simulink model "PMSM_ud_uq_regelung_BackUp"  (R2014b)
settings: Solver=ode4  StartTime=0.0  StopTime=0.2  FixedStep=5e-6  RelTol=1e-3
values from neighbouring files (symbols this model uses):
  f = 50    [parameter.mat]
  J = 0.00062    [parameter.mat]
  Ld = 0.000835    [parameter.mat]
  Lq = 0.000835    [parameter.mat]
  n_soll = 3000    [parameter.mat]
  p = 4    [parameter.mat]
  Psi_pm = 0.07147    [parameter.mat]
  R1 = 0.18    [parameter.mat]
settings Model: Creator=benjamin  LastModifiedBy=Benji

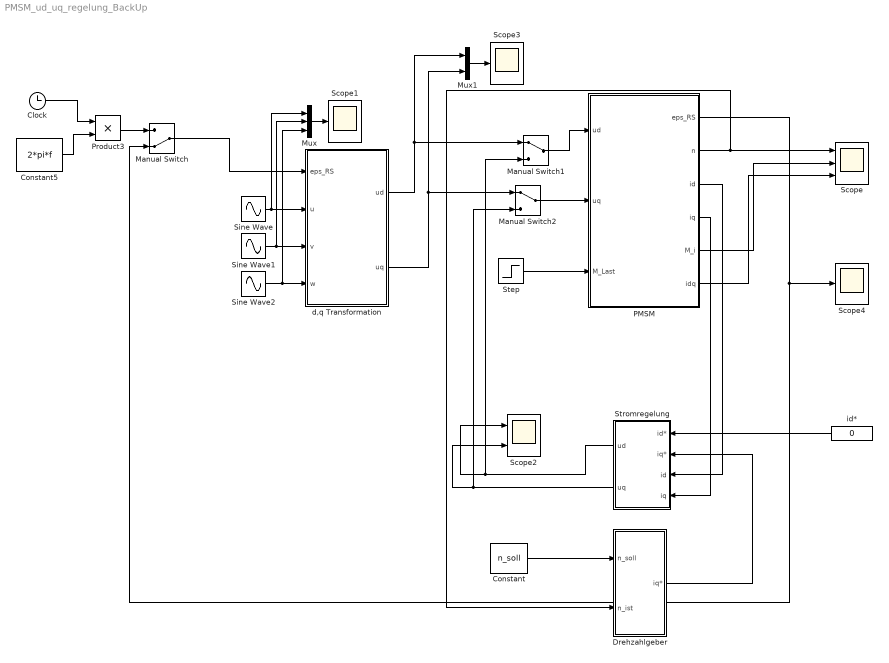
== system PMSM_ud_uq_regelung_BackUp ==
  Clock : Clock
  Constant : Constant  Value=n_soll
  Constant5 : Constant  Value=2*pi*f
  Drehzahlgeber : Subsystem
  Manual Switch : ManualSwitch  CurrentSetting=0
  Manual Switch1 : ManualSwitch
  Manual Switch2 : ManualSwitch
  Mux : Mux  Inputs=3
  Mux1 : Mux  Inputs=2
  PMSM : Subsystem
  Product3 : Product
  Scope : Scope  NumInputPorts=3
      settings: TimeRange=0.0108462013588635  YMin=0~-400~-800  YMax=1200~400~800  SaveName=ScopeData6
  Scope1 : Scope
      settings: TimeRange=0.2  YMin=-25000  YMax=20000
  Scope2 : Scope  NumInputPorts=2
      settings: TimeRange=0.2  YMin=-25000~-400  YMax=20000~400  SaveName=ScopeData2
  Scope3 : Scope
      settings: TimeRange=0.2  YMin=-25000  YMax=20000  SaveName=ScopeData3
  Scope4 : Scope
      settings: TimeRange=0.2  YMin=-25000  YMax=20000  SaveName=ScopeData4
  Sine Wave : Sin  Amplitude=230  Frequency=2*pi*f  SampleTime=0
  Sine Wave1 : Sin  Amplitude=230  Frequency=2*pi*f  Phase=(-2/3)*pi  SampleTime=0
  Sine Wave2 : Sin  Amplitude=230  Frequency=2*pi*f  Phase=(2/3)*pi  SampleTime=0
  Step : Step  Time=0.1  After=40  SampleTime=0
  Stromregelung : Subsystem
  d,q Transformation : Subsystem
  id* : Constant  Value=0
  wires:
  id*/1 -> Stromregelung/1(id*)
  Drehzahlgeber/1(iq*) -> Stromregelung/2(iq*)
  Constant/1 -> Drehzahlgeber/1(n_soll)
  PMSM/2(n) -> Drehzahlgeber/2(n_ist), Scope/1
  PMSM/5(M_i) -> Scope/2
  PMSM/6(idq) -> Scope/3
  Sine Wave/1 -> Mux/1, d,q Transformation/2(u)
  Sine Wave1/1 -> Mux/2, d,q Transformation/3(v)
  Sine Wave2/1 -> Mux/3, d,q Transformation/4(w)
  Mux/1 -> Scope1/1
  Stromregelung/1(ud) -> Scope2/1, Manual Switch1/2
  Stromregelung/2(uq) -> Scope2/2, Manual Switch2/2
  PMSM/3(id) -> Stromregelung/3(id)
  PMSM/4(iq) -> Stromregelung/4(iq)
  Mux1/1 -> Scope3/1
  d,q Transformation/1(ud) -> Manual Switch1/1, Mux1/1
  d,q Transformation/2(uq) -> Manual Switch2/1, Mux1/2
  Clock/1 -> Product3/1
  Constant5/1 -> Product3/2
  Product3/1 -> Manual Switch/1
  Manual Switch/1 -> d,q Transformation/1(eps_RS)
  PMSM/1(eps_RS) -> Scope4/1, Manual Switch/2
  Manual Switch1/1 -> PMSM/1("ud ")
  Manual Switch2/1 -> PMSM/2(uq)
  Step/1 -> PMSM/3(M_Last)

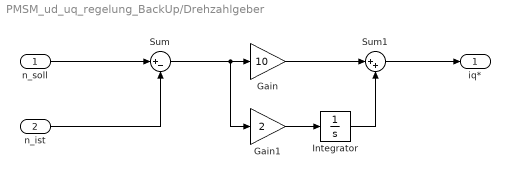
== system PMSM_ud_uq_regelung_BackUp/Drehzahlgeber ==
  n_soll : Inport
  n_ist : Inport  Port=2
  Gain : Gain  Gain=10
  Gain1 : Gain  Gain=2
  Integrator : Integrator
  Sum : Sum  Inputs=|+-
  Sum1 : Sum  Inputs=|++
  iq* : Outport
  wires:
  n_soll/1 -> Sum/1
  n_ist/1 -> Sum/2
  Sum/1 -> Gain1/1, Gain/1
  Gain/1 -> Sum1/1
  Gain1/1 -> Integrator/1
  Integrator/1 -> Sum1/2
  Sum1/1 -> iq*/1

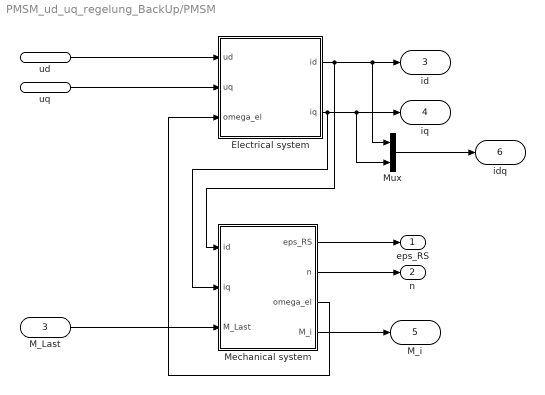
== system PMSM_ud_uq_regelung_BackUp/PMSM ==
  "ud " : Inport
  uq : Inport  Port=2
  M_Last : Inport  Port=3
  Electrical system : Subsystem
  Mechanical system : Subsystem
  Mux : Mux  Inputs=2
  eps_RS : Outport
  n : Outport  Port=2
  id : Outport  Port=3
  iq : Outport  Port=4
  M_i : Outport  Port=5
  idq : Outport  Port=6
  wires:
  Electrical system/1(id) -> Mux/1, id/1, Mechanical system/1(id)
  Electrical system/2(iq) -> Mux/2, iq/1, Mechanical system/2(iq)
  Mechanical system/3(omega_el) -> Electrical system/3(omega_el)
  Mechanical system/1(eps_RS) -> eps_RS/1
  Mechanical system/2(n) -> n/1
  Mechanical system/4(M_i) -> M_i/1
  M_Last/1 -> Mechanical system/3(M_Last)
  uq/1 -> Electrical system/2(uq)
  "ud "/1 -> Electrical system/1(ud)
  Mux/1 -> idq/1

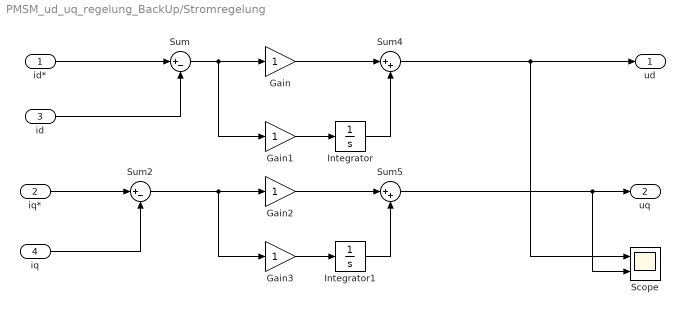
== system PMSM_ud_uq_regelung_BackUp/Stromregelung ==
  id* : Inport
  iq* : Inport  Port=2
  id : Inport  Port=3
  iq : Inport  Port=4
  Gain{,1..3} (4 alike) : Gain
  Integrator : Integrator
  Integrator1 : Integrator
  Scope : Scope  NumInputPorts=2
      settings: TimeRange=5  YMin=-1.3~-5  YMax=0~5
  Sum : Sum  Inputs=|+-
  Sum2 : Sum  Inputs=|+-
  Sum4 : Sum  Inputs=|++
  Sum5 : Sum  Inputs=|++
  ud : Outport
  uq : Outport  Port=2
  wires:
  Sum5/1 -> Scope/2, uq/1
  iq*/1 -> Sum2/1
  id*/1 -> Sum/1
  id/1 -> Sum/2
  iq/1 -> Sum2/2
  Sum4/1 -> ud/1, Scope/1
  Sum/1 -> Gain1/1, Gain/1
  Gain/1 -> Sum4/1
  Gain1/1 -> Integrator/1
  Integrator/1 -> Sum4/2
  Sum2/1 -> Gain3/1, Gain2/1
  Gain2/1 -> Sum5/1
  Gain3/1 -> Integrator1/1
  Integrator1/1 -> Sum5/2

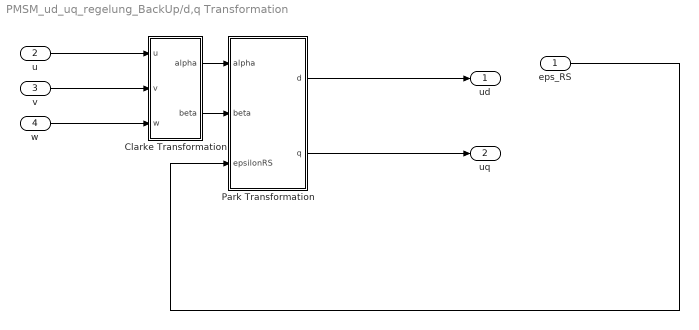
== system PMSM_ud_uq_regelung_BackUp/d,q Transformation ==
  eps_RS : Inport
  u : Inport  Port=2
  v : Inport  Port=3
  w : Inport  Port=4
  Clarke Transformation : Subsystem
  Park Transformation : Subsystem
  ud : Outport
  uq : Outport  Port=2
  wires:
  eps_RS/1 -> Park Transformation/3(epsilonRS)
  Clarke Transformation/1(alpha) -> Park Transformation/1(alpha)
  Clarke Transformation/2(beta) -> Park Transformation/2(beta)
  Park Transformation/1(d) -> ud/1
  Park Transformation/2(q) -> uq/1
  v/1 -> Clarke Transformation/2(v)
  u/1 -> Clarke Transformation/1(u)
  w/1 -> Clarke Transformation/3(w)

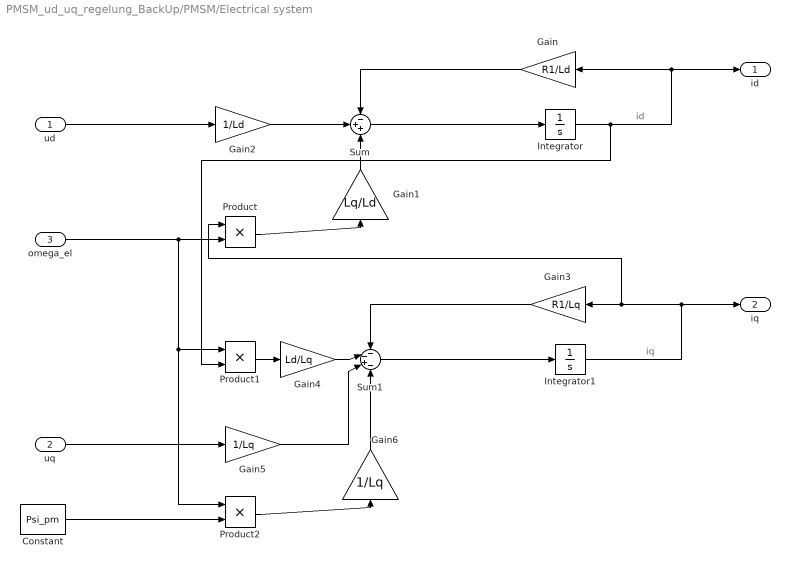
== system PMSM_ud_uq_regelung_BackUp/PMSM/Electrical system ==
  note: id
  note: iq
  ud : Inport
  uq : Inport  Port=2
  omega_el : Inport  Port=3
  Constant : Constant  Value=Psi_pm
  Gain : Gain  Gain=R1/Ld
  Gain1 : Gain  Gain=Lq/Ld
  Gain2 : Gain  Gain=1/Ld
  Gain3 : Gain  Gain=R1/Lq
  Gain4 : Gain  Gain=Ld/Lq
  Gain5 : Gain  Gain=1/Lq
  Gain6 : Gain  Gain=1/Lq
  Integrator : Integrator
  Integrator1 : Integrator
  Product : Product
  Product1 : Product
  Product2 : Product
  Sum : Sum  Inputs=-++
  Sum1 : Sum  Inputs=--+-
  id : Outport
  iq : Outport  Port=2
  wires:
  Sum/1 -> Integrator/1
  Integrator/1 -> Product1/2, Gain/1, id/1
  Gain/1 -> Sum/1
  omega_el/1 -> Product2/1, Product1/1, Product/2
  Gain1/1 -> Sum/3
  Product/1 -> Gain1/1
  ud/1 -> Gain2/1
  Gain2/1 -> Sum/2
  Sum1/1 -> Integrator1/1
  Integrator1/1 -> iq/1, Product/1, Gain3/1
  Gain3/1 -> Sum1/1
  Gain5/1 -> Sum1/3
  Product1/1 -> Gain4/1
  Gain4/1 -> Sum1/2
  uq/1 -> Gain5/1
  Constant/1 -> Product2/2
  Gain6/1 -> Sum1/4
  Product2/1 -> Gain6/1

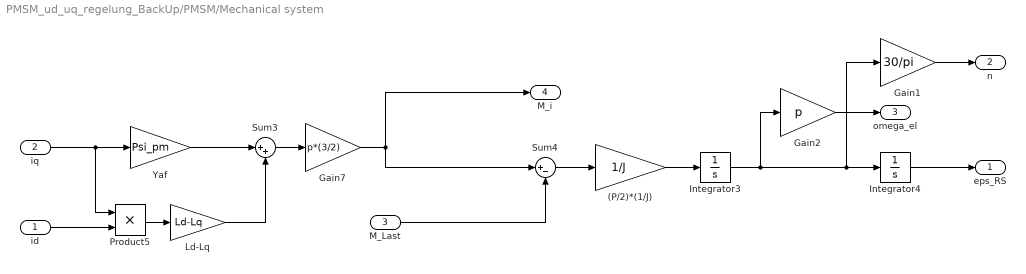
== system PMSM_ud_uq_regelung_BackUp/PMSM/Mechanical system ==
  id : Inport
  iq : Inport  Port=2
  M_Last : Inport  Port=3
  (P/2)*(1/J) : Gain  Gain=1/J
  Gain1 : Gain  Gain=30/pi
  Gain2 : Gain  Gain=p
  Gain7 : Gain  Gain=p*(3/2)
  Integrator3 : Integrator
  Integrator4 : Integrator
  Ld-Lq : Gain  Gain=Ld-Lq
  Product5 : Product  RndMeth=Zero
  Sum3 : Sum  Inputs=|++
  Sum4 : Sum  Inputs=|+-
  Yaf : Gain  Gain=Psi_pm
  eps_RS : Outport
  n : Outport  Port=2
  omega_el : Outport  Port=3
  M_i : Outport  Port=4
  wires:
  Yaf/1 -> Sum3/1
  Sum3/1 -> Gain7/1
  Ld-Lq/1 -> Sum3/2
  Product5/1 -> Ld-Lq/1
  Sum4/1 -> (P/2)*(1/J)/1
  iq/1 -> Product5/1, Yaf/1
  id/1 -> Product5/2
  Gain7/1 -> Sum4/1, M_i/1
  (P/2)*(1/J)/1 -> Integrator3/1
  Integrator4/1 -> eps_RS/1
  Gain1/1 -> n/1
  Integrator3/1 -> Gain1/1, Integrator4/1, Gain2/1
  M_Last/1 -> Sum4/2
  Gain2/1 -> omega_el/1

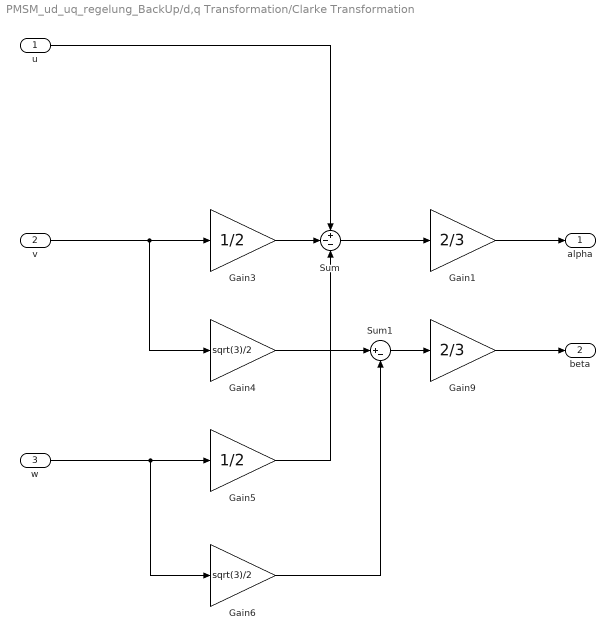
== system PMSM_ud_uq_regelung_BackUp/d,q Transformation/Clarke Transformation ==
  u : Inport
  v : Inport  Port=2
  w : Inport  Port=3
  Gain1 : Gain  Gain=2/3
  Gain3 : Gain  Gain=1/2
  Gain4 : Gain  Gain=sqrt(3)/2
  Gain5 : Gain  Gain=1/2
  Gain6 : Gain  Gain=sqrt(3)/2
  Gain9 : Gain  Gain=2/3
  Sum : Sum  Inputs=+--
  Sum1 : Sum  Inputs=|+-
  alpha : Outport
  beta : Outport  Port=2
  wires:
  Gain5/1 -> Sum/3
  Gain3/1 -> Sum/2
  v/1 -> Gain4/1, Gain3/1
  w/1 -> Gain6/1, Gain5/1
  Gain6/1 -> Sum1/2
  Gain4/1 -> Sum1/1
  Sum/1 -> Gain1/1
  Gain1/1 -> alpha/1
  u/1 -> Sum/1
  Sum1/1 -> Gain9/1
  Gain9/1 -> beta/1

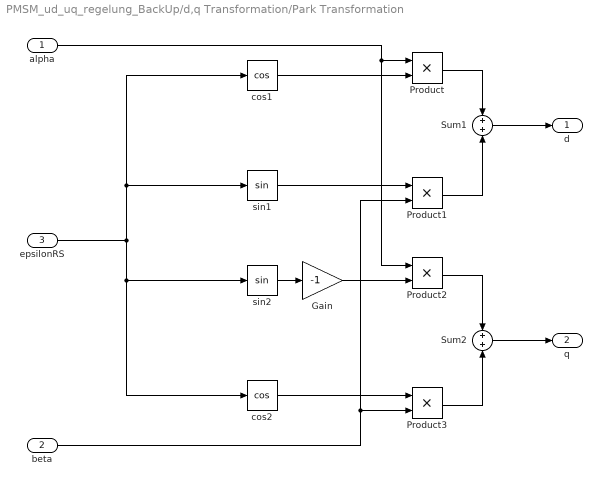
== system PMSM_ud_uq_regelung_BackUp/d,q Transformation/Park Transformation ==
  alpha : Inport
  beta : Inport  Port=2
  epsilonRS : Inport  Port=3
  Gain : Gain  Gain=-1
  Product{,1..3} (4 alike) : Product
  Sum1 : Sum
  Sum2 : Sum
  cos1 : Trigonometry  Operator=cos
  cos2 : Trigonometry  Operator=cos
  sin1 : Trigonometry
  sin2 : Trigonometry
  d : Outport
  q : Outport  Port=2
  wires:
  Sum2/1 -> q/1
  Product2/1 -> Sum2/1
  Product1/1 -> Sum1/2
  epsilonRS/1 -> sin1/1, cos1/1, sin2/1, cos2/1
  cos1/1 -> Product/2
  alpha/1 -> Product2/1, Product/1
  Sum1/1 -> d/1
  cos2/1 -> Product3/1
  beta/1 -> Product3/2, Product1/2
  Product/1 -> Sum1/1
  sin1/1 -> Product1/1
  Product3/1 -> Sum2/2
  sin2/1 -> Gain/1
  Gain/1 -> Product2/2
